simulink library "autopilot_plane"  (Simulink 7.6)
settings: Solver=ode45  SolverMode=SingleTasking  StartTime=0.0  StopTime=10.0  RelTol=1e-3
values from neighbouring files (symbols this model uses):
  a = 2.5348    [f14_digital_data.mat]    (also in f14dat_digital.m; sanim.m = size(vert); sanim3dof.m = size(vert))
  b = 64.13    [f14_digital_data.mat]    (also in f14dat_digital.m)
  Md = -6.8847    [f14_digital_data.mat]    (also in f14dat_digital.m)
  Mq = -0.6571    [f14_digital_data.mat]    (also in f14dat_digital.m)
  Mw = -0.00592    [f14_digital_data.mat]    (also in f14dat_digital.m)
  Swg = 3    [f14_digital_data.mat]    (also in f14dat_digital.m)
  Ta = 0.05    [f14_digital_data.mat]    (also in f14dat_digital.m)
  Ts = 0.1    [f14_digital_data.mat]    (also in f14dat_digital.m)
  Uo = 689.4    [f14_digital_data.mat]    (also in f14dat_digital.m)
  Vto = 690.4    [f14_digital_data.mat]    (also in f14dat_digital.m)
  Zd = -63.9979    [f14_digital_data.mat]    (also in f14dat_digital.m)
  Zw = -0.6385    [f14_digital_data.mat]    (also in f14dat_digital.m)
undefined symbols (not defined in the file or in its folder): alt_ic
libraries: simulink x1
settings Model: Creator=The MathWorks Inc.  ExtModeAutoUpdateStatusClock=off

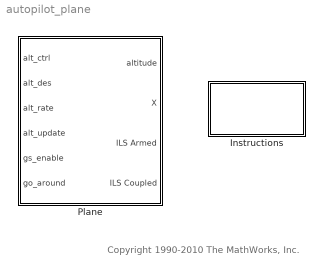
== system autopilot_plane ==
  note: Copyright 1990-2010 The MathWorks, Inc.
  Instructions : Subsystem
      mask Display: disp('Flight\nInstructions\n(double-click)')
  Plane : Subsystem

== system autopilot_plane/Instructions ==
  note: The autopilot is preconfigured for landing.
      |
      | To simulate a landing, set the initial altitude to 1200 by double clicking
      | the setup landing block.  Make sure that the ILS signal is ON and the reset
      | signal is OFF.  The controller will automatically enter glide-slope control when the
      | plane initially crosses the target glide-slope line.  The simulation stop time is set
      | to 150 seconds.
      |
      | To simulate a set point change you should first adjust the desired altitude
      | and vertical speed and then set the update signal to ON to force the new set
      | point into the controller.  The control logic will automatically transition to the
      | altitude climb mode and back to the altitude hold mode as needed.  Change
      | the simulation stop time to 'inf' for an indefinite flight time.

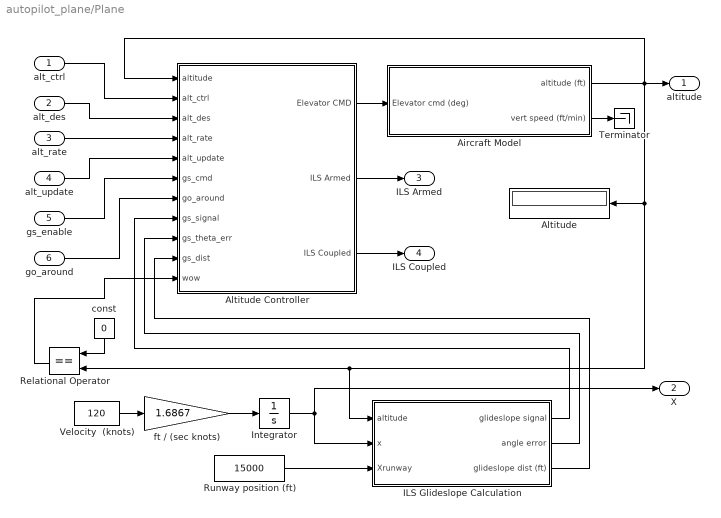
== system autopilot_plane/Plane ==
  alt_ctrl : Inport
  alt_des : Inport  Port=2
  alt_rate : Inport  Port=3
  alt_update : Inport  Port=4
  gs_enable : Inport  Port=5
  go_around : Inport  Port=6
  Aircraft Model : Subsystem
  Altitude : Display
  Altitude Controller : Subsystem
  ILS Glideslope Calculation : Subsystem
  Integrator : Integrator
  Relational Operator : RelationalOperator  Operator===  InputSameDT=on
  Runway position (ft) : Constant  Value=15000
  Terminator : Terminator
  Velocity  (knots) : Constant  Value=120
  const : Constant  Value=0
  ft / (sec knots) : Gain  Gain=1.6867  SaturateOnIntegerOverflow=on  OutDataTypeStr=Inherit: Same as input  ParamDataTypeStr=Inherit: Same as input
  altitude : Outport
  X : Outport  Port=2
  ILS Armed : Outport  Port=3
  ILS Coupled : Outport  Port=4
  wires:
  Altitude Controller/1(Elevator CMD) -> Aircraft Model/1(Elevator cmd (deg))
  Aircraft Model/1(altitude (ft)) -> altitude/1, Altitude Controller/1(altitude), Altitude/1, ILS Glideslope Calculation/1(altitude), Relational Operator/2
  ft / (sec knots)/1 -> Integrator/1
  Velocity  (knots)/1 -> ft / (sec knots)/1
  Integrator/1 -> ILS Glideslope Calculation/2(x), X/1
  Runway position (ft)/1 -> ILS Glideslope Calculation/3(Xrunway)
  ILS Glideslope Calculation/2(angle error) -> Altitude Controller/9(gs_theta_err)
  ILS Glideslope Calculation/3(glideslope dist (ft)) -> Altitude Controller/10(gs_dist)
  ILS Glideslope Calculation/1(glideslope signal) -> Altitude Controller/8(gs_signal)
  Aircraft Model/2(vert speed (ft/min)) -> Terminator/1
  alt_ctrl/1 -> Altitude Controller/2(alt_ctrl)
  alt_des/1 -> Altitude Controller/3(alt_des)
  alt_rate/1 -> Altitude Controller/4(alt_rate)
  alt_update/1 -> Altitude Controller/5(alt_update)
  gs_enable/1 -> Altitude Controller/6(gs_cmd)
  go_around/1 -> Altitude Controller/7(go_around)
  Altitude Controller/2(ILS Armed) -> ILS Armed/1
  Altitude Controller/3(ILS Coupled) -> ILS Coupled/1
  Relational Operator/1 -> Altitude Controller/11(wow)
  const/1 -> Relational Operator/1

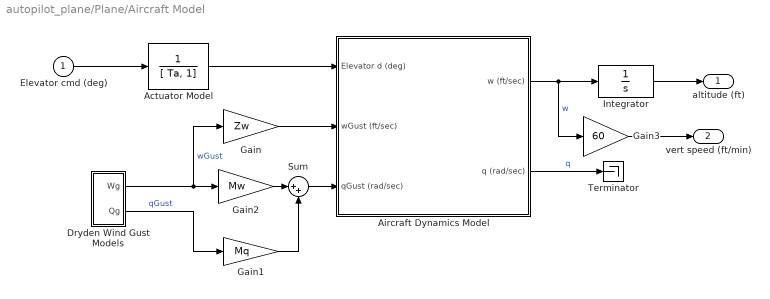
== system autopilot_plane/Plane/Aircraft Model ==
  Elevator cmd (deg) : Inport
  Actuator Model : TransferFcn  Denominator=[ Ta, 1]
  Aircraft Dynamics Model : Subsystem
  Dryden Wind Gust Models : Subsystem
  Gain : Gain  Gain=Zw  SaturateOnIntegerOverflow=on  OutDataTypeStr=Inherit: Same as input  ParamDataTypeStr=Inherit: Same as input
  Gain1 : Gain  Gain=Mq  SaturateOnIntegerOverflow=on  OutDataTypeStr=Inherit: Same as input  ParamDataTypeStr=Inherit: Same as input
  Gain2 : Gain  Gain=Mw  SaturateOnIntegerOverflow=on  OutDataTypeStr=Inherit: Same as input  ParamDataTypeStr=Inherit: Same as input
  Gain3 : Gain  Gain=60  SaturateOnIntegerOverflow=on  OutDataTypeStr=Inherit: Same as input  ParamDataTypeStr=Inherit: Same as input
  Integrator : Integrator  InitialCondition=alt_ic  LimitOutput=on  LowerSaturationLimit=0
  Sum : Sum  Inputs=|++  SaturateOnIntegerOverflow=on  InputSameDT=on  OutDataTypeStr=Inherit: Same as first input
  Terminator : Terminator
  altitude (ft) : Outport
  vert speed (ft/min) : Outport  Port=2
  wires:
  Gain3/1 -> vert speed (ft/min)/1
  Integrator/1 -> altitude (ft)/1
  Aircraft Dynamics Model/2(q (rad/sec)) -> Terminator/1  "q"
  Elevator cmd (deg)/1 -> Actuator Model/1
  Aircraft Dynamics Model/1(w (ft/sec)) -> Gain3/1, Integrator/1  "w"
  Actuator Model/1 -> Aircraft Dynamics Model/1(Elevator d (deg))
  Gain1/1 -> Sum/2
  Dryden Wind Gust Models/1(Wg) -> Gain2/1, Gain/1  "wGust"
  Dryden Wind Gust Models/2(Qg) -> Gain1/1  "qGust"
  Gain2/1 -> Sum/1
  Gain/1 -> Aircraft Dynamics Model/2(wGust (ft/sec))
  Sum/1 -> Aircraft Dynamics Model/3(qGust (rad/sec))

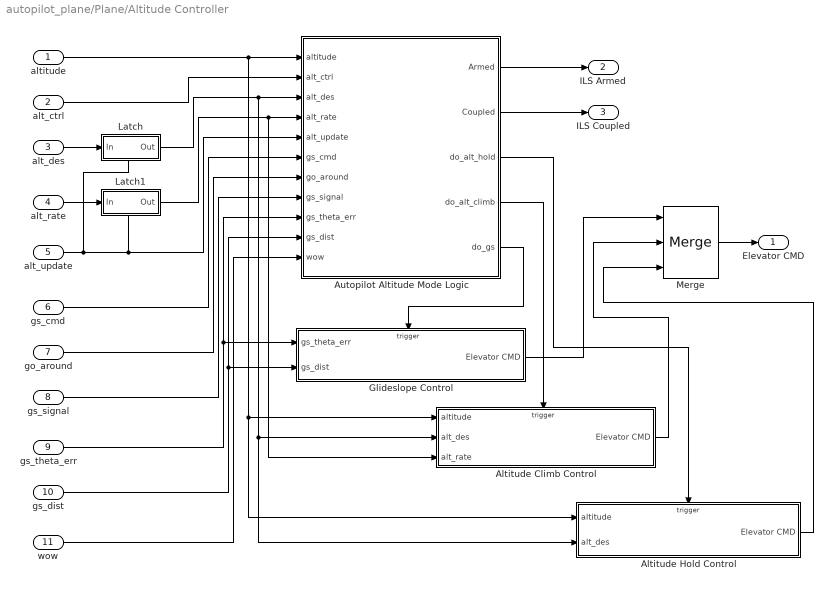
== system autopilot_plane/Plane/Altitude Controller ==
  altitude : Inport  SampleTime=Ts
  alt_ctrl : Inport  Port=2  SampleTime=Ts
  alt_des : Inport  Port=3  SampleTime=Ts
  alt_rate : Inport  Port=4  SampleTime=Ts
  alt_update : Inport  Port=5  SampleTime=Ts
  gs_cmd : Inport  Port=6  SampleTime=Ts
  go_around : Inport  Port=7  SampleTime=Ts
  gs_signal : Inport  Port=8  SampleTime=Ts
  gs_theta_err : Inport  Port=9  SampleTime=Ts
  gs_dist : Inport  Port=10  SampleTime=Ts
  wow : Inport  Port=11  SampleTime=Ts
  Altitude Climb Control : Subsystem  TreatAsAtomicUnit=on
  Altitude Hold Control : Subsystem  TreatAsAtomicUnit=on
  Autopilot Altitude Mode Logic : Stateflow chart  TreatAsAtomicUnit=on
  Glideslope Control : Subsystem  TreatAsAtomicUnit=on
  Latch : Subsystem  TreatAsAtomicUnit=on
      settings: RTWSystemCode=Inline
  Latch1 : Subsystem  TreatAsAtomicUnit=on
      settings: RTWSystemCode=Inline
  Merge : Merge  Inputs=3
  Elevator CMD : Outport
  ILS Armed : Outport  Port=2
  ILS Coupled : Outport  Port=3
  wires:
  Autopilot Altitude Mode Logic/5(do_gs) -> Glideslope Control/Trigger
  Autopilot Altitude Mode Logic/4(do_alt_climb) -> Altitude Climb Control/Trigger
  Autopilot Altitude Mode Logic/3(do_alt_hold) -> Altitude Hold Control/Trigger
  Glideslope Control/1(Elevator CMD) -> Merge/1
  Altitude Climb Control/1(Elevator CMD) -> Merge/2
  Altitude Hold Control/1(Elevator CMD) -> Merge/3
  Merge/1 -> Elevator CMD/1
  altitude/1 -> Altitude Hold Control/1(altitude), Altitude Climb Control/1(altitude), Autopilot Altitude Mode Logic/1(altitude)
  alt_ctrl/1 -> Autopilot Altitude Mode Logic/2(alt_ctrl)
  alt_update/1 -> Latch1/Enable, Autopilot Altitude Mode Logic/5(alt_update), Latch/Enable
  gs_cmd/1 -> Autopilot Altitude Mode Logic/6(gs_cmd)
  go_around/1 -> Autopilot Altitude Mode Logic/7(go_around)
  gs_signal/1 -> Autopilot Altitude Mode Logic/8(gs_signal)
  gs_theta_err/1 -> Glideslope Control/1(gs_theta_err), Autopilot Altitude Mode Logic/9(gs_theta_err)
  gs_dist/1 -> Glideslope Control/2(gs_dist), Autopilot Altitude Mode Logic/10(gs_dist)
  Autopilot Altitude Mode Logic/1(Armed) -> ILS Armed/1
  alt_des/1 -> Latch/1(In)
  Latch/1(Out) -> Altitude Hold Control/2(alt_des), Altitude Climb Control/2(alt_des), Autopilot Altitude Mode Logic/3(alt_des)
  alt_rate/1 -> Latch1/1(In)
  Latch1/1(Out) -> Altitude Climb Control/3(alt_rate), Autopilot Altitude Mode Logic/4(alt_rate)
  wow/1 -> Autopilot Altitude Mode Logic/11(wow)
  Autopilot Altitude Mode Logic/2(Coupled) -> ILS Coupled/1

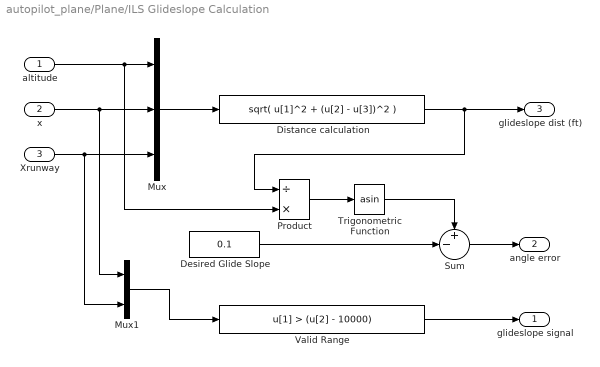
== system autopilot_plane/Plane/ILS Glideslope Calculation ==
  altitude : Inport
  x : Inport  Port=2
  Xrunway : Inport  Port=3
  Desired Glide Slope : Constant  Value=0.1
  Distance calculation : Fcn  Expr=sqrt( u[1]^2 + (u[2] - u[3])^2 )
  Mux : Mux  Inputs=3
  Mux1 : Mux  Inputs=2
  Product : Product  Inputs=/*  SaturateOnIntegerOverflow=on  InputSameDT=on  OutDataTypeStr=Inherit: Same as first input
  Sum : Sum  Inputs=+-|  SaturateOnIntegerOverflow=on  InputSameDT=on  OutDataTypeStr=Inherit: Same as first input
  Trigonometric Function : Trigonometry  Operator=asin
  Valid Range : Fcn  Expr=u[1] > (u[2] - 10000)
  glideslope signal : Outport
  angle error : Outport  Port=2
  glideslope dist (ft) : Outport  Port=3
  wires:
  Mux/1 -> Distance calculation/1
  altitude/1 -> Mux/1, Product/2
  Distance calculation/1 -> glideslope dist (ft)/1, Product/1
  x/1 -> Mux/2, Mux1/1
  Xrunway/1 -> Mux/3, Mux1/2
  Desired Glide Slope/1 -> Sum/2
  Sum/1 -> angle error/1
  Product/1 -> Trigonometric Function/1
  Trigonometric Function/1 -> Sum/1
  Mux1/1 -> Valid Range/1
  Valid Range/1 -> glideslope signal/1

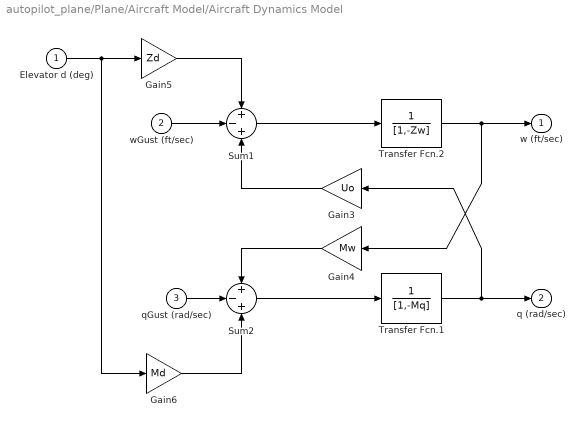
== system autopilot_plane/Plane/Aircraft Model/Aircraft Dynamics Model ==
  Elevator d (deg) : Inport
  wGust (ft/sec) : Inport  Port=2
  qGust (rad/sec) : Inport  Port=3
  Gain3 : Gain  Gain=Uo  SaturateOnIntegerOverflow=on  OutDataTypeStr=Inherit: Same as input  ParamDataTypeStr=Inherit: Same as input
  Gain4 : Gain  Gain=Mw  SaturateOnIntegerOverflow=on  OutDataTypeStr=Inherit: Same as input  ParamDataTypeStr=Inherit: Same as input
  Gain5 : Gain  Gain=Zd  SaturateOnIntegerOverflow=on  OutDataTypeStr=Inherit: Same as input  ParamDataTypeStr=Inherit: Same as input
  Gain6 : Gain  Gain=Md  SaturateOnIntegerOverflow=on  OutDataTypeStr=Inherit: Same as input  ParamDataTypeStr=Inherit: Same as input
  Sum1 : Sum  Inputs=+-+  SaturateOnIntegerOverflow=on  InputSameDT=on  OutDataTypeStr=Inherit: Same as first input
  Sum2 : Sum  Inputs=+-+  SaturateOnIntegerOverflow=on  InputSameDT=on  OutDataTypeStr=Inherit: Same as first input
  Transfer Fcn.1 : TransferFcn  Denominator=[1,-Mq]
  Transfer Fcn.2 : TransferFcn  Denominator=[1,-Zw]
  w (ft/sec) : Outport  InitialOutput=0
  q (rad/sec) : Outport  Port=2  InitialOutput=0
  wires:
  Transfer Fcn.2/1 -> w (ft/sec)/1, Gain4/1
  Transfer Fcn.1/1 -> q (rad/sec)/1, Gain3/1
  Gain6/1 -> Sum2/3
  Gain5/1 -> Sum1/1
  Gain3/1 -> Sum1/3
  qGust (rad/sec)/1 -> Sum2/2
  Sum2/1 -> Transfer Fcn.1/1
  Sum1/1 -> Transfer Fcn.2/1
  Gain4/1 -> Sum2/1
  wGust (ft/sec)/1 -> Sum1/2
  Elevator d (deg)/1 -> Gain5/1, Gain6/1

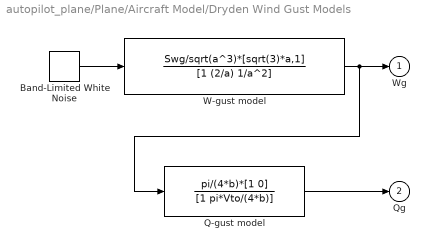
== system autopilot_plane/Plane/Aircraft Model/Dryden Wind Gust Models ==
  Band-Limited White Noise : simulink/Sources/Band-Limited White Noise  Cov=1  Ts=0.2  seed=[23341]
  Q-gust model : TransferFcn  Numerator=pi/(4*b)*[1 0]  Denominator=[1 pi*Vto/(4*b)]
  W-gust model : TransferFcn  Numerator=Swg/sqrt(a^3)*[sqrt(3)*a,1]  Denominator=[1 (2/a) 1/a^2]
  Wg : Outport  InitialOutput=0
  Qg : Outport  Port=2  InitialOutput=0
  wires:
  Band-Limited White Noise/1 -> W-gust model/1
  Q-gust model/1 -> Qg/1
  W-gust model/1 -> Wg/1, Q-gust model/1

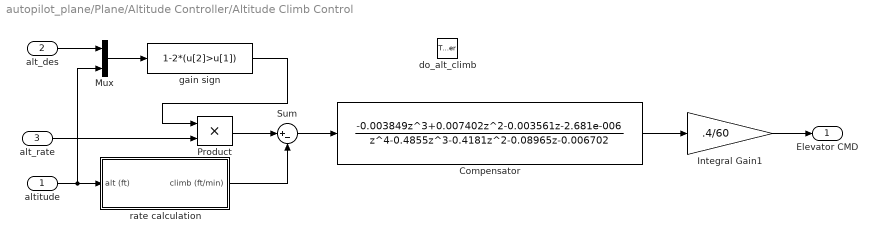
== system autopilot_plane/Plane/Altitude Controller/Altitude Climb Control ==
  altitude : Inport
  alt_des : Inport  Port=2
  alt_rate : Inport  Port=3
  do_alt_climb : TriggerPort  TriggerType=function-call
  Compensator : DiscreteTransferFcn  Numerator="[-0.003849   0.007402  -0.003561 -2.681e-006]"  Denominator="[1 -0.4855  -0.4181 -0.08965  -0.006702]"  SampleTime=-1
  Integral Gain1 : Gain  Gain=.4/60  SaturateOnIntegerOverflow=on  OutDataTypeStr=Inherit: Same as input  ParamDataTypeStr=Inherit: Same as input
  Mux : Mux  Inputs=2
  Product : Product  SaturateOnIntegerOverflow=on  InputSameDT=on  OutDataTypeStr=Inherit: Same as first input
  Sum : Sum  Inputs=|+-  SaturateOnIntegerOverflow=on  InputSameDT=on  OutDataTypeStr=Inherit: Same as first input
  gain sign : Fcn  Expr=1-2*(u[2]>u[1])
  rate calculation : Subsystem
  Elevator CMD : Outport
  wires:
  Sum/1 -> Compensator/1
  rate calculation/1(climb (ft/min)) -> Sum/2
  altitude/1 -> rate calculation/1(alt (ft)), Mux/2
  alt_des/1 -> Mux/1
  Mux/1 -> gain sign/1
  Product/1 -> Sum/1
  alt_rate/1 -> Product/2
  gain sign/1 -> Product/1
  Compensator/1 -> Integral Gain1/1
  Integral Gain1/1 -> Elevator CMD/1

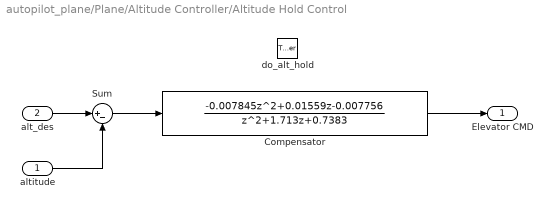
== system autopilot_plane/Plane/Altitude Controller/Altitude Hold Control ==
  altitude : Inport
  alt_des : Inport  Port=2
  do_alt_hold : TriggerPort  TriggerType=function-call
  Compensator : DiscreteTransferFcn  Numerator="[-0.007845  0.01559 -0.007756]"  Denominator="[1 1.713  0.7383]"  SampleTime=-1
  Sum : Sum  Inputs=|+-  SaturateOnIntegerOverflow=on  InputSameDT=on  OutDataTypeStr=Inherit: Same as first input
  Elevator CMD : Outport
  wires:
  alt_des/1 -> Sum/1
  altitude/1 -> Sum/2
  Compensator/1 -> Elevator CMD/1
  Sum/1 -> Compensator/1

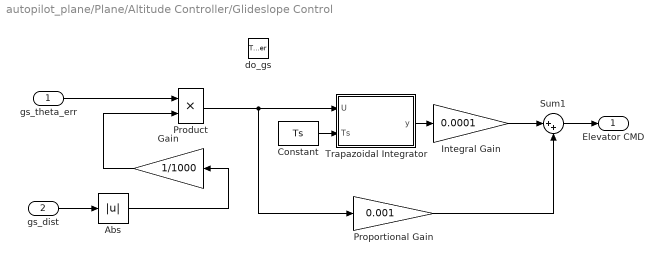
== system autopilot_plane/Plane/Altitude Controller/Glideslope Control ==
  gs_theta_err : Inport
  gs_dist : Inport  Port=2
  do_gs : TriggerPort  TriggerType=function-call
  Abs : Abs  SaturateOnIntegerOverflow=on
  Constant : Constant  Value=Ts
  Gain : Gain  Gain=1/1000  SaturateOnIntegerOverflow=on  OutDataTypeStr=Inherit: Same as input  ParamDataTypeStr=Inherit: Same as input
  Integral Gain : Gain  Gain=0.0001  SaturateOnIntegerOverflow=on  OutDataTypeStr=Inherit: Same as input  ParamDataTypeStr=Inherit: Same as input
  Product : Product  SaturateOnIntegerOverflow=on  InputSameDT=on  OutDataTypeStr=Inherit: Same as first input
  Proportional Gain : Gain  Gain=0.001  SaturateOnIntegerOverflow=on  OutDataTypeStr=Inherit: Same as input  ParamDataTypeStr=Inherit: Same as input
  Sum1 : Sum  Inputs=|++  SaturateOnIntegerOverflow=on  InputSameDT=on  OutDataTypeStr=Inherit: Same as first input
  Trapazoidal Integrator : Subsystem
      mask Type: No Time Trapazoid Integrator
      mask Description: Discrete-time integrator with no dependence on absolute time.  U is the input value and Ts is the discrete sample time.
      mask Display:
      | disp(sprintf('T(z+1)\n-----\n2(z-1)'))
      | port_label('input',1,'U');
      | port_label('input',2,'Ts');
  Elevator CMD : Outport
  wires:
  Sum1/1 -> Elevator CMD/1
  Integral Gain/1 -> Sum1/1
  Proportional Gain/1 -> Sum1/2
  Trapazoidal Integrator/1(y) -> Integral Gain/1
  Product/1 -> Proportional Gain/1, Trapazoidal Integrator/1(U)
  gs_theta_err/1 -> Product/1
  Gain/1 -> Product/2
  Abs/1 -> Gain/1
  gs_dist/1 -> Abs/1
  Constant/1 -> Trapazoidal Integrator/2(Ts)

== system autopilot_plane/Plane/Altitude Controller/Latch ==
  In : Inport
  Enable : EnablePort
  Out : Outport  InitialOutput=alt_ic
  wires:
  In/1 -> Out/1

== system autopilot_plane/Plane/Altitude Controller/Latch1 ==
  In : Inport
  Enable : EnablePort
  Out : Outport  InitialOutput=10000
  wires:
  In/1 -> Out/1

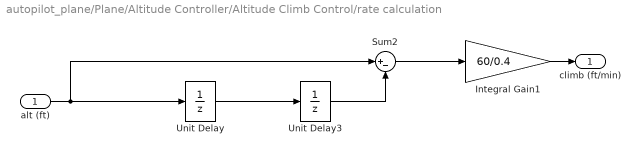
== system autopilot_plane/Plane/Altitude Controller/Altitude Climb Control/rate calculation ==
  alt (ft) : Inport
  Integral Gain1 : Gain  Gain=60/0.4  SaturateOnIntegerOverflow=on  OutDataTypeStr=Inherit: Same as input  ParamDataTypeStr=Inherit: Same as input
  Sum2 : Sum  Inputs=|+-  SaturateOnIntegerOverflow=on  InputSameDT=on  OutDataTypeStr=Inherit: Same as first input
  Unit Delay : UnitDelay  X0=10000  SampleTime=-1
  Unit Delay3 : UnitDelay  X0=10000  SampleTime=-1
  climb (ft/min) : Outport
  wires:
  Unit Delay/1 -> Unit Delay3/1
  alt (ft)/1 -> Unit Delay/1, Sum2/1
  Unit Delay3/1 -> Sum2/2
  Sum2/1 -> Integral Gain1/1
  Integral Gain1/1 -> climb (ft/min)/1

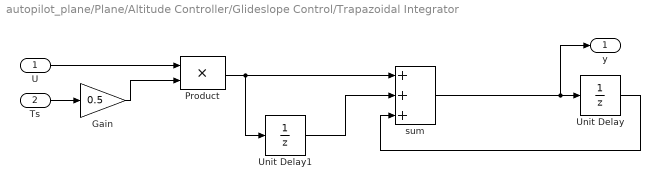
== system autopilot_plane/Plane/Altitude Controller/Glideslope Control/Trapazoidal Integrator ==
  U : Inport
  Ts : Inport  Port=2
  Gain : Gain  Gain=0.5  OutDataTypeStr=Inherit: Same as input  ParamDataTypeStr=Inherit: Same as input
  Product : Product  InputSameDT=on  OutDataTypeStr=Inherit: Same as first input
  Unit Delay : UnitDelay  SampleTime=-1
  Unit Delay1 : UnitDelay  SampleTime=-1
  sum : Sum  Inputs=+++  InputSameDT=on  OutDataTypeStr=Inherit: Same as first input
  y : Outport
  wires:
  Ts/1 -> Gain/1
  Gain/1 -> Product/2
  U/1 -> Product/1
  Unit Delay/1 -> sum/3
  sum/1 -> y/1, Unit Delay/1
  Unit Delay1/1 -> sum/2
  Product/1 -> Unit Delay1/1, sum/1

== stateflow chart Plane/Altitude Controller/Autopilot Altitude Mode Logic ==
  settings: updateMethod=DISCRETE  sampleTime=Ts
  state out = alt_capture() [function]
    (default) -> (junction 19) : {out = abs(altitude - alt_des) < 30*Ts*(alt_rate / 60);}
  state GS [parallel]
    settings: executionOrder=1
    state Off
    state Active
      state Armed
      state Coupled /du: do_gs;
        state Around
        state Norm
        (default) -> Norm
        Norm -> Around : [go_around]
      Armed -> Coupled /du: do_gs; : [gs_coupled()]
      (default) -> Armed
    GS.Active -> Off : [~gs_cmd | ...
        |  ~gs_signal | wow]
    (default) -> Off
    Off -> GS.Active : [gs_cmd & ...
        | gs_signal & ~wow]
  state out = gs_coupled() [function]
    (default) -> (junction 18) : {out = gs_dist<10000 & gs_theta_err>0;}
  note: Glideslope
  state Altitude [parallel]
    settings: executionOrder=2
    state Disabled
    state Active
      state Climb_Rate
        du: do_alt_climb;
      state Hold
        du: do_alt_hold;
      Hold -> Climb_Rate : [abs(altitude-alt_des) >1500]
      Climb_Rate -> Hold : [alt_capture()]
    Disabled -> Hold : [alt_ctrl & ~wow & ...
        | ~in(GS.Active.Coupled)]
    (default) -> Disabled
    Altitude.Active -> Disabled : [in(GS.Active.Coupled) | ...
        | ~alt_ctrl | wow]
  data: out function_output double; out function_output double; altitude input double; alt_ctrl input boolean; alt_des input double; alt_rate input double; alt_update input boolean; gs_cmd input boolean; go_around input boolean; gs_signal input double; gs_theta_err input double; gs_dist input double; Ts parameter double =0.2; Armed output unknown; Coupled output unknown; wow input boolean
  events: do_alt_hold output FUNCTION_CALL_EVENT; do_alt_climb output FUNCTION_CALL_EVENT; do_gs output FUNCTION_CALL_EVENT
